simulink model "GeneratePulseFcn"  (R2022a)
settings: Solver=FixedStepAuto  StartTime=0.0  StopTime=Inf  FixedStep=SAMPLING_TIME  RelTol=1e-3
libraries: simulink x1
Description:
  | % Copyright 2019 The MathWorks, Inc.
settings Model: DataDictionary=Parameters.sldd  EnableAccessToBaseWorkspace=off  Creator=sdupertu  LastModifiedBy=sebas
settings SolverCC: AlgebraicLoopSolver=TrustRegion
settings DataIOCC: SaveOutput=off  SaveTime=off
settings OptimizationCC: DefaultParameterBehavior=Inlined  EnhancedBackFolding=on  PassReuseOutputArgsAs=Individual arguments  OptimizeBlockOrder=speed  DifferentSizesBufferReuse=on  OptimizationCustomize=off  EfficientTunableParamExpr=on
settings DebuggingCC: ParameterTunabilityLossMsg=error  UnconnectedInputMsg=warning  UnconnectedOutputMsg=warning  UnconnectedLineMsg=warning  PregeneratedLibrarySubsystemCodeDiagnostic=none  SFMachineParentedDataDiag=warning  ArithmeticOperatorsInVariantConditions=warning
settings ModelReferenceCC: EnableParallelModelReferenceBuilds=on
settings SFSimCC: SimUseLocalCustomCode=off  MATLABDynamicMemAlloc=off  CustomCodeUndefinedFunction=UseInterfaceOnly
settings RTWCC: SystemTargetFile=ert.tlc  TemplateMakefile=ert_default_tmf  GenerateReport=on  RTWUseLocalCustomCode=off  IncludeHyperlinkInReport=on  LaunchReport=on  GenerateTraceInfo=on  GenerateTraceReport=on  GenerateTraceReportSl=on  GenerateTraceReportSf=on  GenerateTraceReportEml=on  GenerateWebview=on  GenerateCodeMetricsReport=on  DLArmComputeVersion=19.05
settings CodeAppCC: ForceParamTrailComments=on  IgnoreCustomStorageClasses=off  MaxIdLength=61  OperatorAnnotations=on  SimulinkDataObjDesc=on  SFDataObjDesc=on  InsertBlockDesc=on
settings ERTTargetCC: TargetLangStandard=C99 (ISO)  GenerateSampleERTMain=on  InlinedParameterPlacement=NonHierarchical  ERTCustomFileTemplate=example_file_process.tlc

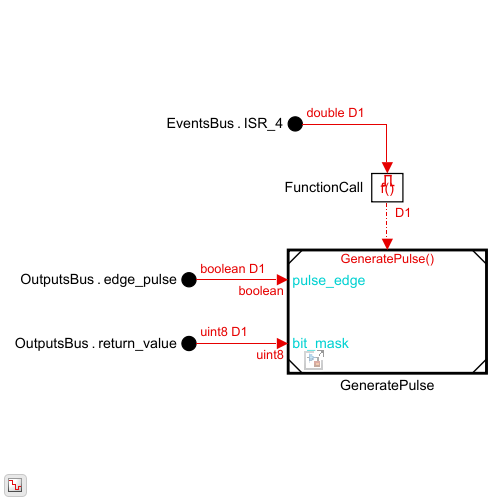
[thumbnail: Simulink's stored preview of the top-level diagram]
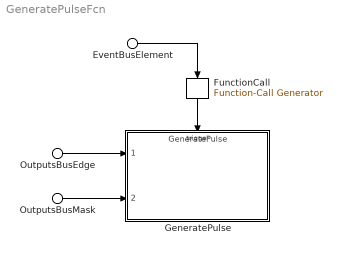
== system GeneratePulseFcn ==
  OutputsBusEdge : Inport  PortName=OutputsBus  Element=edge_pulse
  OutputsBusMask : Inport  PortName=OutputsBus  Element=return_value
  EventBusElement : Inport  Port=2  PortName=EventsBus  Element=ISR_4
  FunctionCall : simulink/Ports & Subsystems/Function-Call Generator  sample_time=1  numberOfIterations=1  DisallowWideOutput=off  ShowEnablePort=on
  GeneratePulse : ModelReference  ModelNameDialog=GeneratePulse.slx  SimulationMode=Normal  ModelReferenceVersion=6.2  TriggerPortName=call  TriggerPortTriggerType=function-call  TriggerPortStatesWhenEnabling=held
  wires:
  OutputsBusEdge/1 -> GeneratePulse/1
  FunctionCall/1 -> GeneratePulse/Trigger
  EventBusElement/1 -> FunctionCall/1
  OutputsBusMask/1 -> GeneratePulse/2
